simulink model "single2uintX"  (R2014b)
settings: Solver=FixedStepDiscrete  StartTime=0.0  StopTime=1  FixedStep=1  RelTol=1e-3
libraries: simulink x10
settings Model: DataTypeOverride=Single  DataTypeOverrideAppliesTo=Floating-point  Creator=rchladny  LastModifiedBy=rchladny

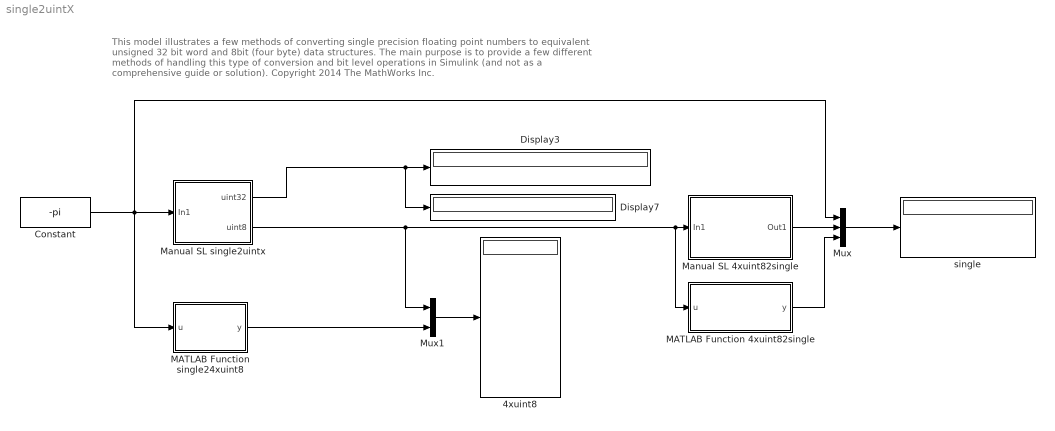
== system single2uintX ==
  note: This model illustrates a few methods of converting single precision floating point numbers to equivalent unsigned 32 bit word and 8bit (four byte) data structures.
      | The main purpose is to provide a few different methods of handling this type of conversion and bit level operations in Simulink (and not as a comprehensive guide or solution).
      |
      | Copyright 2014 The MathWorks Inc.
  4xuint8 : Display
  Constant : Constant  Value=-pi  OutDataTypeStr=single
  Display3 : Display
      settings: Format=binary (Stored Integer)
  Display7 : Display
  MATLAB Function 4xuint82single : MATLAB Function  TreatAsAtomicUnit=on
  MATLAB Function single24xuint8 : MATLAB Function  TreatAsAtomicUnit=on
  Manual SL 4xuint82single : Subsystem
  Manual SL single2uintx : Subsystem
  Mux : Mux  Inputs=3
  Mux1 : Mux  Inputs=2
  single : Display
  wires:
  Constant/1 -> Mux/1, MATLAB Function single24xuint8/1(u), Manual SL single2uintx/1(In1)
  MATLAB Function single24xuint8/1(y) -> Mux1/2
  Manual SL single2uintx/2(uint8) -> Mux1/1, MATLAB Function 4xuint82single/1(u), Manual SL 4xuint82single/1(In1)
  MATLAB Function 4xuint82single/1(y) -> Mux/3
  Manual SL 4xuint82single/1(Out1) -> Mux/2
  Manual SL single2uintx/1(uint32) -> Display7/1, Display3/1
  Mux/1 -> single/1
  Mux1/1 -> 4xuint8/1

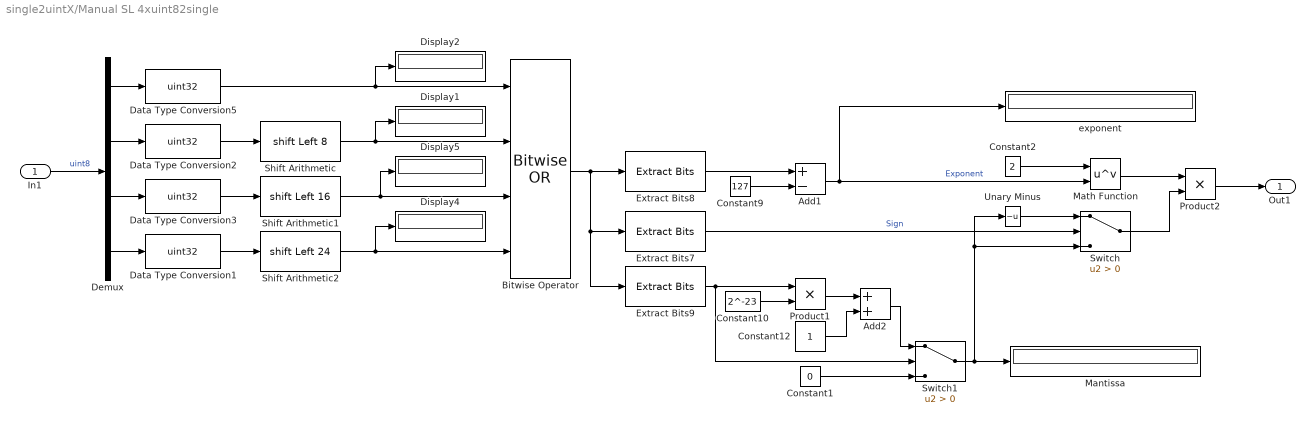
== system single2uintX/Manual SL 4xuint82single ==
  In1 : Inport
  Add1 : Sum  Inputs=+-  OutDataTypeStr=single
  Add2 : Sum  OutDataTypeStr=single
  Bitwise Operator : simulink/Logic and Bit Operations/Bitwise Operator  logicop=OR  UseBitMask=off  NumInputPorts=4  BitMask=bin2dec('11011001')  BitMaskRealWorld=Stored Integer
  Constant1 : Constant  Value=0  OutDataTypeStr=single
  Constant10 : Constant  Value=2^-23  OutDataTypeStr=single
  Constant12 : Constant  OutDataTypeStr=single
  Constant2 : Constant  Value=2  OutDataTypeStr=single
  Constant9 : Constant  Value=127  OutDataTypeStr=uint8
  Data Type Conversion{1..3,5} (4 alike) : DataTypeConversion  OutDataTypeStr=uint32  ConvertRealWorld=Stored Integer (SI)
  Demux : Demux
  Display{1..2,4..5} (4 alike) : Display
  Extract Bits7 : simulink/Logic and Bit Operations/Extract Bits  bitsToExtract=Range of bits  numBits=8  bitIdxRange=31  outScalingMode=Treat bit field as an integer
  Extract Bits8 : simulink/Logic and Bit Operations/Extract Bits  bitsToExtract=Range of bits  numBits=8  bitIdxRange=[23 30]  outScalingMode=Treat bit field as an integer
  Extract Bits9 : simulink/Logic and Bit Operations/Extract Bits  bitsToExtract=Range of bits  numBits=8  bitIdxRange=[0 22]  outScalingMode=Treat bit field as an integer
  Mantissa : Display
  Math Function : Math  Operator=pow  OutputSignalType=real  SaturateOnIntegerOverflow=on
  Product1 : Product  Inputs=**
  Product2 : Product  Inputs=**
  Shift Arithmetic : ArithShift  BitShiftNumber=8  BitShiftDirection=Left
  Shift Arithmetic1 : ArithShift  BitShiftNumber=16  BitShiftDirection=Left
  Shift Arithmetic2 : ArithShift  BitShiftNumber=24  BitShiftDirection=Left
  Switch : Switch  Criteria=u2 > Threshold
  Switch1 : Switch  Criteria=u2 > Threshold
  Unary Minus : UnaryMinus
  exponent : Display
  Out1 : Outport
  wires:
  Product2/1 -> Out1/1
  Extract Bits7/1 -> Switch/2  "Sign"
  Extract Bits8/1 -> Add1/1
  Extract Bits9/1 -> Switch1/2, Product1/1
  Constant10/1 -> Product1/2
  Product1/1 -> Add2/1
  Math Function/1 -> Product2/1
  Unary Minus/1 -> Switch/1
  Add1/1 -> Math Function/2, exponent/1  "Exponent"
  Add2/1 -> Switch1/1
  Switch/1 -> Product2/2
  Constant9/1 -> Add1/2
  Bitwise Operator/1 -> Extract Bits7/1, Extract Bits9/1, Extract Bits8/1
  Constant12/1 -> Add2/2
  Constant2/1 -> Math Function/1
  Constant1/1 -> Switch1/3
  Switch1/1 -> Mantissa/1, Unary Minus/1, Switch/3
  Demux/3 -> Data Type Conversion3/1
  Demux/4 -> Data Type Conversion1/1
  Shift Arithmetic/1 -> Bitwise Operator/2, Display1/1
  Demux/2 -> Data Type Conversion2/1
  Shift Arithmetic1/1 -> Bitwise Operator/3, Display5/1
  Shift Arithmetic2/1 -> Bitwise Operator/4, Display4/1
  Data Type Conversion2/1 -> Shift Arithmetic/1
  Data Type Conversion3/1 -> Shift Arithmetic1/1
  Demux/1 -> Data Type Conversion5/1
  Data Type Conversion5/1 -> Bitwise Operator/1, Display2/1
  In1/1 -> Demux/1  "uint8"
  Data Type Conversion1/1 -> Shift Arithmetic2/1

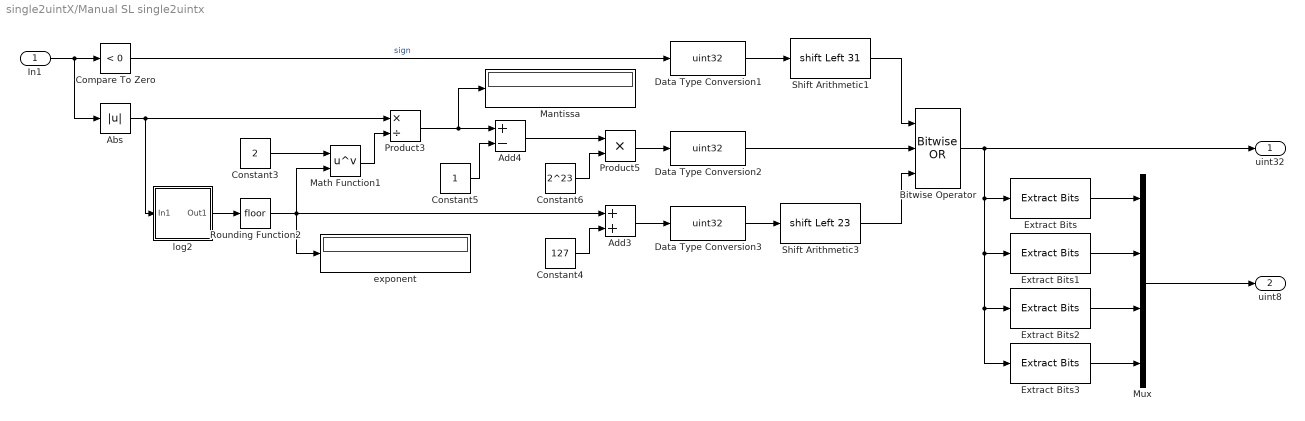
== system single2uintX/Manual SL single2uintx ==
  In1 : Inport
  Abs : Abs
  Add3 : Sum  OutDataTypeStr=single
  Add4 : Sum  Inputs=+-  OutDataTypeStr=single
  Bitwise Operator : simulink/Logic and Bit Operations/Bitwise Operator  logicop=OR  UseBitMask=off  NumInputPorts=3  BitMask=bin2dec('11011001')  BitMaskRealWorld=Stored Integer
  Compare To Zero : simulink/Logic and Bit Operations/Compare To Zero  relop=<  OutDataTypeStr=boolean
  Constant3 : Constant  Value=2  OutDataTypeStr=single
  Constant4 : Constant  Value=127  OutDataTypeStr=uint8
  Constant5 : Constant  OutDataTypeStr=single
  Constant6 : Constant  Value=2^23  OutDataTypeStr=single
  Data Type Conversion1 : DataTypeConversion  OutDataTypeStr=uint32
  Data Type Conversion2 : DataTypeConversion  OutDataTypeStr=uint32
  Data Type Conversion3 : DataTypeConversion  OutDataTypeStr=uint32
  Extract Bits : simulink/Logic and Bit Operations/Extract Bits  bitsToExtract=Range of bits  numBits=8  bitIdxRange=[0 7]  outScalingMode=Treat bit field as an integer
  Extract Bits1 : simulink/Logic and Bit Operations/Extract Bits  bitsToExtract=Range of bits  numBits=8  bitIdxRange=[8 15]  outScalingMode=Treat bit field as an integer
  Extract Bits2 : simulink/Logic and Bit Operations/Extract Bits  bitsToExtract=Range of bits  numBits=8  bitIdxRange=[16 23]  outScalingMode=Treat bit field as an integer
  Extract Bits3 : simulink/Logic and Bit Operations/Extract Bits  bitsToExtract=Range of bits  numBits=8  bitIdxRange=[24 31]  outScalingMode=Treat bit field as an integer
  Mantissa : Display
  Math Function1 : Math  Operator=pow  OutputSignalType=real  SaturateOnIntegerOverflow=on
  Mux : Mux
  Product3 : Product  Inputs=*/
  Product5 : Product  Inputs=**
  Rounding Function2 : Rounding
  Shift Arithmetic1 : ArithShift  BitShiftNumber=31  BitShiftDirection=Left
  Shift Arithmetic3 : ArithShift  BitShiftNumber=23  BitShiftDirection=Left
  exponent : Display
  log2 : Subsystem
  uint32 : Outport
  uint8 : Outport  Port=2
  wires:
  In1/1 -> Abs/1, Compare To Zero/1
  Data Type Conversion1/1 -> Shift Arithmetic1/1
  Compare To Zero/1 -> Data Type Conversion1/1  "sign"
  Shift Arithmetic1/1 -> Bitwise Operator/1
  Abs/1 -> log2/1(In1), Product3/1
  Constant3/1 -> Math Function1/1
  Math Function1/1 -> Product3/2
  Product3/1 -> Mantissa/1, Add4/1
  Rounding Function2/1 -> exponent/1, Add3/1, Math Function1/2
  Constant4/1 -> Add3/2
  Add3/1 -> Data Type Conversion3/1
  Data Type Conversion3/1 -> Shift Arithmetic3/1
  Shift Arithmetic3/1 -> Bitwise Operator/3
  Constant5/1 -> Add4/2
  Add4/1 -> Product5/1
  Product5/1 -> Data Type Conversion2/1
  Data Type Conversion2/1 -> Bitwise Operator/2
  log2/1(Out1) -> Rounding Function2/1
  Constant6/1 -> Product5/2
  Extract Bits/1 -> Mux/1
  Extract Bits1/1 -> Mux/2
  Extract Bits2/1 -> Mux/3
  Extract Bits3/1 -> Mux/4
  Mux/1 -> uint8/1
  Bitwise Operator/1 -> Extract Bits2/1, Extract Bits3/1, Extract Bits1/1, Extract Bits/1, uint32/1

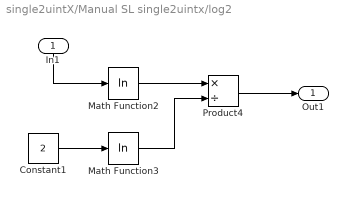
== system single2uintX/Manual SL single2uintx/log2 ==
  In1 : Inport
  Constant1 : Constant  Value=2  OutDataTypeStr=single
  Math Function2 : Math  Operator=log  OutputSignalType=real  SaturateOnIntegerOverflow=on
  Math Function3 : Math  Operator=log  OutputSignalType=real  SaturateOnIntegerOverflow=on
  Product4 : Product  Inputs=*/
  Out1 : Outport
  wires:
  In1/1 -> Math Function2/1
  Product4/1 -> Out1/1
  Constant1/1 -> Math Function3/1
  Math Function2/1 -> Product4/1
  Math Function3/1 -> Product4/2

== matlab function single2uintX/MATLAB Function single24xuint8 ==
  data: u input single size=1; y output uint8
function y = fcn(u)
%#codegen

y = typecast(single(u),'uint8');

== matlab function single2uintX/MATLAB Function 4xuint82single ==
  data: u input uint8; y output
function y = fcn(u)
%#codegen

y = typecast(u,'single');
